simulink model "control_system_observer"  (R2022a)
settings: Solver=FixedStepDiscrete  StartTime=t3(1)  StopTime=t3(end)  FixedStep=Ts  RelTol=1e-3
undefined symbols (not defined in the file): A, B, C, D, L, Ts
settings Model: Creator=iande  LastModifiedBy=delg
settings SolverCC: ZeroCrossControl=DisableAll

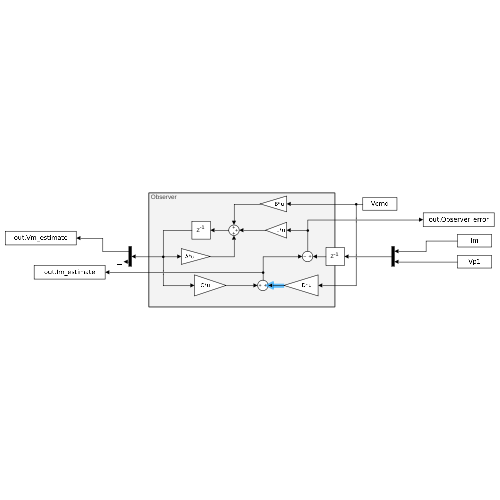
[thumbnail: Simulink's stored preview of the top-level diagram]
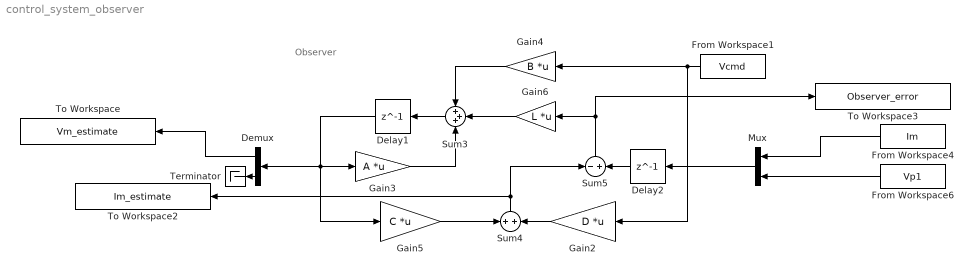
== system control_system_observer ==
  note: Observer
  Delay1 : Delay  DelayLength=1  InitialCondition=0  SampleTime=Ts
  Delay2 : Delay  DelayLength=1  InitialCondition=0  SampleTime=Ts
  Demux : Demux  Outputs=2
  From Workspace1 : FromWorkspace  VariableName=Vcmd  SampleTime=Ts
  From Workspace4 : FromWorkspace  VariableName=Im  SampleTime=Ts
  From Workspace6 : FromWorkspace  VariableName=Vp1  SampleTime=Ts
  Gain2 : Gain  Gain=D  Multiplication=Matrix(K*u)
  Gain3 : Gain  Gain=A  Multiplication=Matrix(K*u)
  Gain4 : Gain  Gain=B  Multiplication=Matrix(K*u)
  Gain5 : Gain  Gain=C  Multiplication=Matrix(K*u)
  Gain6 : Gain  Gain=L  Multiplication=Matrix(K*u)
  Mux : Mux  Inputs=2
  Sum3 : Sum  Inputs=+++
  Sum4 : Sum
  Sum5 : Sum  Inputs=-+
  Terminator : Terminator
  To Workspace : ToWorkspace  VariableName=Vm_estimate  SaveFormat=Timeseries  SampleTime=Ts
  To Workspace2 : ToWorkspace  VariableName=Im_estimate  SaveFormat=Timeseries  SampleTime=Ts
  To Workspace3 : ToWorkspace  VariableName=Observer_error  SaveFormat=Timeseries  SampleTime=Ts
  wires:
  Sum5/1 -> To Workspace3/1, Gain6/1
  Gain2/1 -> Sum4/2
  Sum4/1 -> Sum5/1, To Workspace2/1
  Gain4/1 -> Sum3/1
  Gain3/1 -> Sum3/3
  Gain6/1 -> Sum3/2
  Gain5/1 -> Sum4/1
  Sum3/1 -> Delay1/1
  Delay1/1 -> Gain3/1, Demux/1, Gain5/1
  Delay2/1 -> Sum5/2
  Demux/1 -> To Workspace/1
  Demux/2 -> Terminator/1
  Mux/1 -> Delay2/1
  From Workspace4/1 -> Mux/1
  From Workspace6/1 -> Mux/2
  From Workspace1/1 -> Gain4/1, Gain2/1
